simulink model "validity"  (R2021b)
settings: Solver=FixedStepAuto  StartTime=0.0  StopTime=10.0  RelTol=1e-3
undefined symbols (not defined in the file): sldvsubsys
libraries: sldvlib x6, simulink x1
settings Model: Creator=marco  LastModifiedBy=angelo
settings ConfigComp: DVMode=PropertyProving  DVMaxProcessTime=14400  DVTestSuiteOptimization=Auto  DVDetectOutOfBounds=on  DVMaxViolationSteps=5  DVModelReferenceHarness=on

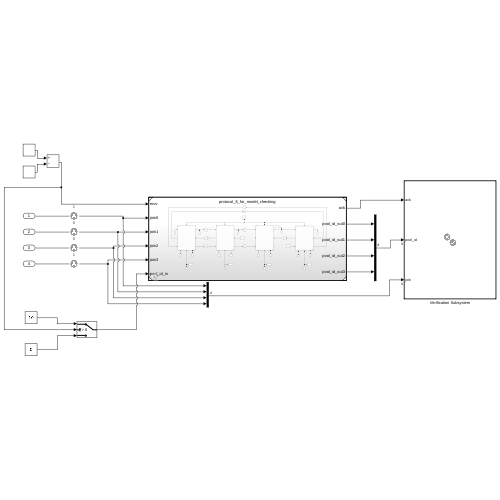
[thumbnail: Simulink's stored preview of the top-level diagram]
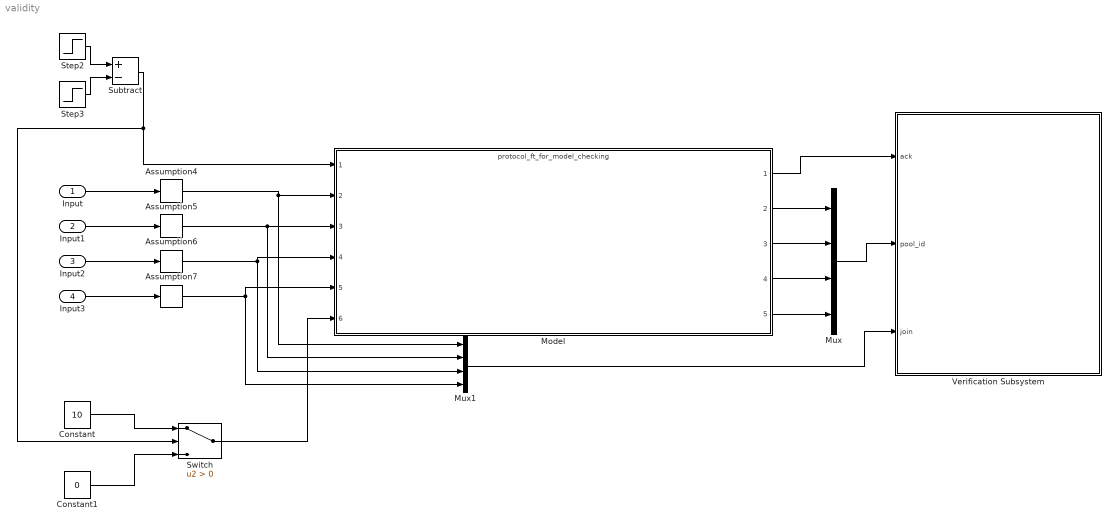
== system validity ==
  Input : Inport
  Input1 : Inport  Port=2
  Input2 : Inport  Port=3
  Input3 : Inport  Port=4
  Assumption4 : sldvlib/Objectives and Constraints/Assumption  enabled=on  customAVTBlockType=Assumption  intervals=1  initial=off  dispValues=on  outEnabled=on
      settings: AttributesFormatString=%<intervals>  SourceProductBaseCode=SL
  Assumption5 : sldvlib/Objectives and Constraints/Assumption  enabled=on  customAVTBlockType=Assumption  intervals=0  initial=off  dispValues=on  outEnabled=on
      settings: AttributesFormatString=%<intervals>  SourceProductBaseCode=SL
  Assumption6 : sldvlib/Objectives and Constraints/Assumption  enabled=on  customAVTBlockType=Assumption  intervals=0  initial=off  dispValues=on  outEnabled=on
      settings: AttributesFormatString=%<intervals>  SourceProductBaseCode=SL
  Assumption7 : sldvlib/Objectives and Constraints/Assumption  enabled=on  customAVTBlockType=Assumption  intervals=1  initial=off  dispValues=on  outEnabled=on
      settings: AttributesFormatString=%<intervals>  SourceProductBaseCode=SL
  Constant : Constant  Value=10
  Constant1 : Constant  Value=0
  Model : ModelReference  ModelNameDialog=protocol_ft_for_model_checking.slx  SimulationMode=Normal  ModelReferenceVersion=1.121
  Mux : Mux
  Mux1 : Mux
  Step2 : Step  SampleTime=.2
  Step3 : Step  Time=1.2  SampleTime=.2
  Subtract : Sum  Inputs=+-
  Switch : Switch  Criteria=u2 > Threshold
  Verification Subsystem : Subsystem  Tag=VerificationSubsystem  DisableCoverage=on  LoadFcn=sldvsubsys('check')  TreatAsAtomicUnit=on  SimViewingDevice=on  mask(VerificationSubsystem){}
      mask init:
      | sldvsubsys('maskInit');
      settings: CopyFcn=sldvsubsys('copy');  OpenFcn=open_system(gcb,'force');
      settings: PreSaveFcn=|
      | set_param(gcb,'SimViewingDevice','on');
      | sldvsubsys('check');
      mask Help: helpview(fullfile(docroot,'toolbox','sldv','sldv.map'),'verificationsubsystem')
      mask Display: image(imread('sldvicon_versubsys.png','BackGroundColor',[1 1 1]),'center');
  wires:
  Mux/1 -> Verification Subsystem/2(pool_id)
  Step3/1 -> Subtract/2
  Step2/1 -> Subtract/1
  Subtract/1 -> Model/1, Switch/2
  Model/2 -> Mux/1
  Model/3 -> Mux/2
  Model/4 -> Mux/3
  Model/5 -> Mux/4
  Model/1 -> Verification Subsystem/1(ack)
  Input/1 -> Assumption4/1
  Input1/1 -> Assumption5/1
  Input2/1 -> Assumption6/1
  Input3/1 -> Assumption7/1
  Mux1/1 -> Verification Subsystem/3(join)
  Assumption4/1 -> Mux1/1, Model/2
  Assumption5/1 -> Mux1/2, Model/3
  Assumption6/1 -> Mux1/3, Model/4
  Assumption7/1 -> Mux1/4, Model/5
  Constant/1 -> Switch/1
  Constant1/1 -> Switch/3
  Switch/1 -> Model/6

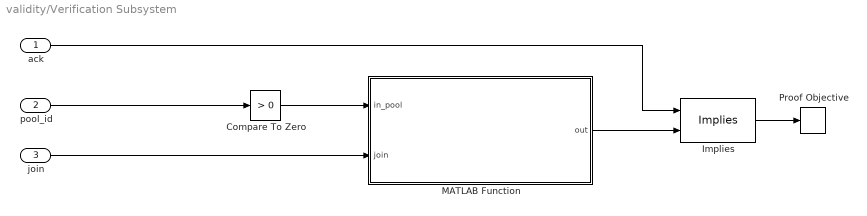
== system validity/Verification Subsystem ==
  ack : Inport
  pool_id : Inport  Port=2
  join : Inport  Port=3
  Compare To Zero : simulink/Logic and Bit Operations/Compare To Zero  relop=>  OutDataTypeStr=boolean
  Implies : sldvlib/Verification Utilities/Implies
      settings: SourceProductBaseCode=SL
  MATLAB Function : MATLAB Function  TreatAsAtomicUnit=on
  Proof Objective : sldvlib/Objectives and Constraints/Proof Objective  enabled=on  customAVTBlockType=Proof Objective  intervals=true  dispValues=on  outEnabled=off  enableStopSim=off
      settings: AttributesFormatString=%<intervals>  SourceProductBaseCode=SL
  wires:
  join/1 -> MATLAB Function/2(join)
  pool_id/1 -> Compare To Zero/1
  ack/1 -> Implies/1
  Implies/1 -> Proof Objective/1
  MATLAB Function/1(out) -> Implies/2
  Compare To Zero/1 -> MATLAB Function/1(in_pool)

== matlab function validity/Verification Subsystem/MATLAB Function ==
  data: in_pool input; join input; out output
function out = validity(in_pool, join)
    out = all((in_pool & join) == in_pool);
end
